simulink model "modules"  (R2017a)
settings: Solver=ode4  StartTime=0.0  StopTime=time_stop  FixedStep=time_step  RelTol=1e-3
values from neighbouring files (symbols this model uses):
  psi = state(3)    [PSVobstacleShip_class.m]    (also in PSVvessel_class.m = obj.eta(3); PsiReferenceModel_class.m = obj.desired_psi_vector; SBMPC_PSVvessel_class.m = obj.eta(3))
undefined symbols (not defined in the file or in its folder): beta, Delta_guidance, Delta_matrix, eta_initial, initial_desired_psi_vector, initial_desired_u_vector, initial_next_waypoint_indexes, initial_obstacle_ship_states, initial_obstacle_ship_states_dot, initial_reference_psi_vector, initial_reference_u_vector, initial_SBMPC_desired_psi_vector, initial_SBMPC_desired_u_vector, initial_SBMPC_next_waypoint_indexes, initial_SBMPC_obstacle_ship_states, initial_SBMPC_obstacle_ship_states_dot, initial_SBMPC_reference_psi_vector, initial_SBMPC_reference_u_vector, initial_SBMPC_x_d_psi_matrix, initial_SBMPC_x_d_u_matrix, initial_state, initial_x_d_psi_matrix, initial_x_d_u_matrix, K_sway, K_yaw, Kp_feedback_linearization, kp_heading, Nmax, nu_initial, num_obs_ship_waypoints, num_prediction_time_steps, number_of_control_behaviors, number_of_obstacle_ships, number_of_SBMPC_obstacle_ships, obs_speed_between_waypoints, obstacle_waypoint_matrix, Omega_matrix, own_ship_reference_psi_init, own_ship_reference_speed, Psi_init, radius_of_acceptance, SBMPC_obs_speed_between_waypoints, SBMPC_obstacle_waypoint_matrix, seconds_between_prediction, state_vector_init, T, T_k_surge, T_k_sway, T_k_yaw, T_s, T_waypoints, time_step, tsamp, U, U_init, V_init, waypoints_obstacle_ships, waypoints_own_ship, Xmax, Ymax
(part 5 of 5)

== matlab function modules/Own-ship/SBMPC /Own-ship trajectory prediction/Own ship trajectory prediction ==
  settings: updateMethod=DISCRETE  sampleTime=time_step
  data: t_0 input; T_s parameter; Kp_feedback_linearization parameter; kp_heading parameter; Xmax parameter; Ymax parameter; Nmax parameter; K_sway parameter; K_yaw parameter; T_k_surge parameter; T_k_sway parameter; T_k_yaw parameter; eta_initial input; nu_initial input; T parameter; Delta_matrix parameter; Omega_matrix parameter; waypoints_matrix input; next_waypoint_index input; own_ship_reference_speed parameter; Delta_guidance parameter; radius_of_acceptance parameter; beta parameter; propulsion_commands parameter; heading_angle_offset_commands parameter; seconds_between_prediction parameter; num_prediction_time_steps parameter; own_ship_x_predicted output size=[num_prediction_time_steps, number_of_control_behaviors]; own_ship_y_predicted output size=[num_prediction_time_steps, number_of_control_behaviors]; own_ship_heading_predicted output size=[num_prediction_time_steps, number_of_control_behaviors]; own_ship_u_predicted output size=[num_prediction_time_steps, number_of_control_behaviors]; own_ship_v_predicted output size=[num_prediction_time_steps, number_of_control_behaviors]; number_of_control_behaviors parameter; own_ship_reference_psi_init parameter
function [own_ship_x_predicted, own_ship_y_predicted, own_ship_heading_predicted, own_ship_u_predicted, own_ship_v_predicted  ]   = ownShipTrajectoryPrediction(t_0, T_s, Kp_feedback_linearization, kp_heading, Xmax, Ymax, Nmax, K_sway, K_yaw, T_k_surge, T_k_sway, T_k_yaw, eta_initial, nu_initial, T, Delta_matrix, Omega_matrix, waypoints_matrix, next_waypoint_index, own_ship_reference_speed, Delta_guidance, radius_of_acceptance, beta, propulsion_commands, heading_angle_offset_commands, seconds_between_prediction, num_prediction_time_steps, number_of_control_behaviors, own_ship_reference_psi_init)  
    %2D zero matrices. One row for each time step in prediction horizon and one column for each control behavior/scenario. 
    own_ship_x_predicted = zeros(num_prediction_time_steps, number_of_control_behaviors);%own_ship_x_predicted_initialization;       
    own_ship_y_predicted = zeros(num_prediction_time_steps, number_of_control_behaviors);%own_ship_y_predicted_initialization;       
    own_ship_heading_predicted = zeros(num_prediction_time_steps, number_of_control_behaviors);%own_ship_heading_predicted_initialization;
    own_ship_u_predicted = zeros(num_prediction_time_steps, number_of_control_behaviors);%own_ship_u_predicted_initialization;
    own_ship_v_predicted = zeros(num_prediction_time_steps, number_of_control_behaviors);%own_ship_v_predicted_initialization;
    
    if (mod(t_0, seconds_between_prediction) == 0)   %only do calculation every "seconds_between_prediction" second.
        psvParameters = coder.load('PSVparameters');
        psvModelParameters = psvParameters.model_config;
        psv_vessel = SBMPC_PSVvessel_class(psvModelParameters, eta_initial, nu_initial, T_s, Kp_feedback_linearization, kp_heading, Xmax, Ymax, Nmax, K_sway, K_yaw, T_k_surge, T_k_sway, T_k_yaw);

        x =  psv_vessel.state(1);
        y =  psv_vessel.state(2);
        vessel_position = [x,y];
        waypointGuidanceObject = SBMPC_waypointGuidance_class(own_ship_reference_psi_init, waypoints_matrix, next_waypoint_index, vessel_position, Delta_guidance, beta, T_s, radius_of_acceptance);              

        scenario_index = 1;  %count for control behaviors
        for Pr = propulsion_commands
            for psi_ca = heading_angle_offset_commands                        
                psv_vessel = psv_vessel.resetPSVState(); %Reset PSV state at start of scenario.
                waypointGuidanceObject = waypointGuidanceObject.resetWaypoints(next_waypoint_index);
                x_d_speed = [nu_initial(1);nu_initial(2);nu_initial(3);0;0;0];
                x_d_heading = [eta_initial(1);eta_initial(2);eta_initial(3);0;0;0;0;0;0];
                for t = 1:num_prediction_time_steps       
                    %Guidance
                    x =  psv_vessel.state(1);
                    y =  psv_vessel.state(2);
                    vessel_position = [x,y];
                    waypointGuidanceObject = waypointGuidanceObject.updateVesselPosition(vessel_position);
                    waypointGuidanceObject = waypointGuidanceObject.updateCurrentWaypoint();                    
                    [waypointGuidanceObject, reference_psi] = waypointGuidanceObject.getReferencePsi();  
                    reference_u = own_ship_reference_speed;

                    %Speed reference model
                    x_d_speed = speedReferenceModel(x_d_speed, reference_u, T_s, Delta_matrix, Omega_matrix);
                    desired_nu = x_d_speed(1:3); 
                    desired_nu(1) = desired_nu(1)*Pr;   %change desired speed in u-direction.
                    
                    x_d_heading = referenceModelPsi(x_d_heading, reference_psi, Omega_matrix, T_s);
                    desired_psi = psi_ca + x_d_heading(3); 
                    

                    [psv_vessel, tau] = psv_vessel.updateStates(desired_psi, desired_nu);       
                    state = psv_vessel.state;                    
                    
                    own_ship_x_predicted(t,scenario_index) = state(1);
                    own_ship_y_predicted(t,scenario_index) = state(2);
                    own_ship_heading_predicted(t,scenario_index) = state(3);
                    own_ship_u_predicted(t,scenario_index) = state(4);
                    own_ship_v_predicted(t,scenario_index) = state(5);
                end %end for
                scenario_index = scenario_index + 1;
            end % end for
        end % end for    
    end %end if    
        
end

== matlab function modules/obstacle ships/Obstacle vessels ==
  data: desired_psi_vector input; desired_u_vector input; obstacle_ships_state_matrix output; X output; Y output; Psi output; U output; V output; R output; Nmax parameter; Ymax parameter; Xmax parameter; kp_heading parameter; Kp_feedback_linearization parameter; initial_obstacle_ship_states parameter; time_step parameter; initial_obstacle_ship_states_dot parameter; number_of_obstacle_ships parameter; K_sway parameter; K_yaw parameter; T_k_yaw parameter; T_k_sway parameter; T_k_surge parameter; state_vector_init parameter; obs_eta output; obs_nu output
function [obstacle_ships_state_matrix, X, Y, Psi, U, V, R, obs_eta, obs_nu] = obstacleVessels(desired_psi_vector, desired_u_vector, Nmax, Ymax, Xmax, kp_heading, Kp_feedback_linearization, initial_obstacle_ship_states, time_step, initial_obstacle_ship_states_dot, number_of_obstacle_ships, K_sway, K_yaw,  T_k_yaw, T_k_sway, T_k_surge, state_vector_init)
    persistent obstacle_ships
    
    if (isempty(obstacle_ships))
        psvParameters = coder.load('PSVparameters');
        psvModelParameters = psvParameters.model_config;
        obstacle_ships = obstacleShips_class(number_of_obstacle_ships, initial_obstacle_ship_states, initial_obstacle_ship_states_dot, desired_psi_vector, desired_u_vector, time_step, psvModelParameters, Kp_feedback_linearization, kp_heading, Xmax, Ymax, Nmax, K_sway, K_yaw, T_k_surge, T_k_sway, T_k_yaw);
    end
    
    
    obstacle_ships = obstacle_ships.updateDesiredSpeedVector(desired_u_vector);
    obstacle_ships = obstacle_ships.updateDesiredPsiVector(desired_psi_vector);    
    obstacle_ships = obstacle_ships.updateObstacleShipsStates();
    
    %each column i in the obstacleShipsStateMatrix is the state [x,y,psi,u,v,r] for obstacle ship number i
    obstacle_ships_state_matrix = obstacle_ships.getObstacleShipsStateMatrix(); 

    
    %column vectors with states. Each element/row r is value for obstacle ship number r
    X = obstacle_ships_state_matrix(1,:);
    Y = obstacle_ships_state_matrix(2,:);
    Psi = obstacle_ships_state_matrix(3,:);
    U = obstacle_ships_state_matrix(4,:);
    V = obstacle_ships_state_matrix(5,:);
    R = obstacle_ships_state_matrix(6,:); 
    obs_eta = [X', Y', Psi'];
    obs_nu  = [U', V', R'];
    
end

== matlab function modules/obstacle ships/find position matrix ==
  data: obstacles_x_position input; position_matrix output; obstacles_y_position input; obstacle_ships_position_matrix_init parameter
function position_matrix = findObstaclePositionMatrix(obstacles_x_position, obstacles_y_position, obstacle_ships_position_matrix_init)
%obstacle positon matrix: %each row r contains x and y position for obstacle ship r

position_matrix = obstacle_ships_position_matrix_init;

position_matrix(:,1) = obstacles_x_position; 
position_matrix(:,2) = obstacles_y_position;
end

== matlab function modules/obstacle ships/guidance /MATLAB Function1 ==
  data: u_vector output; initial_reference_u_vector parameter; next_waypoints_indexes input; obs_speed_between_waypoints parameter; number_of_obstacle_ships parameter
function u_vector = reference_u_vector(initial_reference_u_vector, next_waypoints_indexes, obs_speed_between_waypoints, number_of_obstacle_ships)
    u_vector = initial_reference_u_vector;  %row vector
    for i = 1:number_of_obstacle_ships
        u_vector(i) = obs_speed_between_waypoints(i,next_waypoints_indexes(i)-1);
    end % end for
    
end

== matlab function modules/obstacle ships/guidance /obstacle waypoint guidance ==
  data: obstacle_waypoints input; reference_psi_vector output; state_matrix input; time_step parameter; beta parameter; Delta_guidance parameter; radius_of_acceptance parameter; initial_obstacle_ship_states parameter; number_of_obstacle_ships parameter; initial_reference_psi_vector parameter; initial_next_waypoint_indexes parameter; next_waypoints_indexes output
function [reference_psi_vector, next_waypoints_indexes]  = obstacleWaypointGuidance(obstacle_waypoints, state_matrix, time_step, beta, Delta_guidance, radius_of_acceptance, initial_obstacle_ship_states, number_of_obstacle_ships, initial_reference_psi_vector, initial_next_waypoint_indexes)
    persistent obstaclewaypointGuidanceObject;
    
    if (isempty(obstaclewaypointGuidanceObject))
        obstaclewaypointGuidanceObject = obstacleWaypointGuidance_class(obstacle_waypoints, initial_obstacle_ship_states, Delta_guidance, beta, radius_of_acceptance, time_step, number_of_obstacle_ships, initial_reference_psi_vector, initial_next_waypoint_indexes);
    end
    obstaclewaypointGuidanceObject = obstaclewaypointGuidanceObject.updateObstaclePositions(state_matrix);
    obstaclewaypointGuidanceObject = obstaclewaypointGuidanceObject.updateCurrentWaypoints();
    [obstaclewaypointGuidanceObject, reference_psi_vector] = obstaclewaypointGuidanceObject.getReferencePsiVector();
    next_waypoints_indexes = obstaclewaypointGuidanceObject.getNextWaypointsIndexes();
end

== matlab function modules/obstacle ships/reference model for psi/psi reference model  ==
  data: reference_psi_vector input; desired_psi_vector output; time_step parameter; Delta_matrix parameter; Omega_matrix parameter; initial_reference_psi_vector parameter; number_of_obstacle_ships parameter; initial_desired_psi_vector parameter; initial_x_d_psi_matrix parameter
function desired_psi_vector = obstacleShipsReferenceModelPsi(reference_psi_vector,time_step, Delta_matrix, Omega_matrix, initial_reference_psi_vector,number_of_obstacle_ships,initial_desired_psi_vector, initial_x_d_psi_matrix)

persistent psi_reference_model;

if (isempty(psi_reference_model))
   psi_reference_model = PsiReferenceModel_class(number_of_obstacle_ships, initial_reference_psi_vector, initial_desired_psi_vector, initial_x_d_psi_matrix, Omega_matrix, Delta_matrix, time_step); 
end

psi_reference_model = psi_reference_model.updateReferencePsi(reference_psi_vector);
[psi_reference_model, desired_psi_vector]  = psi_reference_model.updateDesiredPsi();
end

== matlab function modules/obstacle ships/reference model for u/MATLAB Function1 ==
  data: desired_u_vector output; reference_u_vetor input; number_of_obstacle_ships parameter; initial_reference_u_vector parameter; initial_desired_u_vector parameter; initial_x_d_u_matrix parameter; Omega_matrix parameter; Delta_matrix parameter; time_step parameter
function desired_u_vector  = fcn(reference_u_vetor, number_of_obstacle_ships, initial_reference_u_vector, initial_desired_u_vector, initial_x_d_u_matrix, Omega_matrix, Delta_matrix, time_step)
persistent u_reference_model;



if (isempty(u_reference_model))
    u_reference_model = uReferenceModel_class(number_of_obstacle_ships, initial_reference_u_vector, initial_desired_u_vector, initial_x_d_u_matrix, Omega_matrix, Delta_matrix, time_step);
end

u_reference_model = u_reference_model.updateReferenceU(reference_u_vetor);
[u_reference_model, desired_u_vector] = u_reference_model.updateDesiredU();



end

== matlab function modules/SBMPC obstacle ships/SBMPC using intentions /Combine normal obs and own-ship obs ship data  ==
  settings: updateMethod=DISCRETE  sampleTime=time_step
  data: normal_obstacle_ships_x_predicted input size=[number_of_obstacle_ships, num_prediction_time_steps]; obs_x_predicted output size=[1+number_of_obstacle_ships, num_prediction_time_steps]; normal_obstacle_ships_y_predicted input size=[number_of_obstacle_ships, num_prediction_time_steps]; normal_obstacle_ships_Psi input size=[number_of_obstacle_ships, num_prediction_time_steps]; normal_obstacle_ships_U input size=[number_of_obstacle_ships, num_prediction_time_steps]; normal_obsatcle_ships_V input size=[number_of_obstacle_ships, num_prediction_time_steps]; obs_y_predicted output size=[1+number_of_obstacle_ships, num_prediction_time_steps]; obs_psi output size=[1+number_of_obstacle_ships, num_prediction_time_steps]; obs_u output size=[1+number_of_obstacle_ships, num_prediction_time_steps]; obs_v output size=[1+number_of_obstacle_ships, num_prediction_time_steps]; own_ship_obs_x_predicted input size=[num_prediction_time_steps, 1]; own_ship_obs_y_predicted input size=[num_prediction_time_steps, 1]; own_ship_obs_psi input size=[num_prediction_time_steps, 1]; own_ship_obs_u input size=[num_prediction_time_steps, 1]; own_ship_obs_v input size=[num_prediction_time_steps, 1]
function [obs_x_predicted, obs_y_predicted, obs_psi, obs_u, obs_v] = combineNormalAndOwnShipObstacleShipData(normal_obstacle_ships_x_predicted,  normal_obstacle_ships_y_predicted, normal_obstacle_ships_Psi, normal_obstacle_ships_U, normal_obsatcle_ships_V, own_ship_obs_x_predicted, own_ship_obs_y_predicted, own_ship_obs_psi, own_ship_obs_u, own_ship_obs_v)   
   %Data: own ship data as first element , then all normal obstacles data 
   
    obs_x_predicted = [own_ship_obs_x_predicted'; normal_obstacle_ships_x_predicted ];
    obs_y_predicted = [own_ship_obs_y_predicted'; normal_obstacle_ships_y_predicted ];
    
    obs_psi = [own_ship_obs_psi'; normal_obstacle_ships_Psi ]; 
    obs_u   = [own_ship_obs_u';   normal_obstacle_ships_U   ];
    obs_v   = [own_ship_obs_v';   normal_obsatcle_ships_V   ];
   
end

== matlab function modules/Own-ship/SBMPC /Predict obstacle trajectories/Combine normal and SBMPC obstacle ship data  ==
  data: normal_obstacle_ships_x_predicted input size=[num_prediction_time_steps, number_of_obstacle_ships]; obs_x_predicted output size=[num_prediction_time_steps, total_number_of_obstacle_ships]; normal_obstacle_ships_y_predicted input size=[num_prediction_time_steps, number_of_obstacle_ships]; normal_obstacle_ships_Psi input size=[num_prediction_time_steps, number_of_obstacle_ships]; normal_obstacle_ships_U input size=[num_prediction_time_steps, number_of_obstacle_ships]; normal_obsatcle_ships_V input size=[num_prediction_time_steps, number_of_obstacle_ships]; SBMPC_obstacle_ships_X_predicted input size=[number_of_SBMPC_obstacle_ships,num_prediction_time_steps]; SBMPC_obstacle_ships_Y_predicted input size=[number_of_SBMPC_obstacle_ships,num_prediction_time_steps]; SBMPC_obstacle_ships_Psi input size=[number_of_SBMPC_obstacle_ships,num_prediction_time_steps]; SBMPC_obstacle_ships_U input size=[number_of_SBMPC_obstacle_ships,num_prediction_time_steps]; SBMPC_obstacle_ships_V input size=[number_of_SBMPC_obstacle_ships,num_prediction_time_steps]; obs_y_predicted output size=[num_prediction_time_steps, total_number_of_obstacle_ships]; obs_psi output size=[num_prediction_time_steps, total_number_of_obstacle_ships]; obs_u output size=[num_prediction_time_steps, total_number_of_obstacle_ships]; obs_v output size=[num_prediction_time_steps, total_number_of_obstacle_ships]
function [obs_x_predicted, obs_y_predicted, obs_psi, obs_u, obs_v] = combineNormalAndSBMPCObstacleShipData(normal_obstacle_ships_x_predicted,  normal_obstacle_ships_y_predicted, normal_obstacle_ships_Psi, normal_obstacle_ships_U, normal_obsatcle_ships_V,SBMPC_obstacle_ships_X_predicted, SBMPC_obstacle_ships_Y_predicted, SBMPC_obstacle_ships_Psi, SBMPC_obstacle_ships_U, SBMPC_obstacle_ships_V)   
    
    obs_x_predicted = [normal_obstacle_ships_x_predicted, SBMPC_obstacle_ships_X_predicted'];
    obs_y_predicted = [normal_obstacle_ships_y_predicted, SBMPC_obstacle_ships_Y_predicted'];
    
    obs_psi = [normal_obstacle_ships_Psi, SBMPC_obstacle_ships_Psi']; 
    obs_u   = [normal_obstacle_ships_U, SBMPC_obstacle_ships_U'];
    obs_v   = [normal_obsatcle_ships_V, SBMPC_obstacle_ships_V'];
   
end

== matlab function modules/SBMPC obstacle ships/find SBMPC position matrix ==
  data: obstacles_x_position input; position_matrix output; obstacles_y_position input; SBMPC_obstacle_ships_position_matrix_init parameter
function position_matrix = findSBMPCObstaclePositionMatrix(obstacles_x_position, obstacles_y_position, SBMPC_obstacle_ships_position_matrix_init)
%obstacle positon matrix: %each row r contains x and y position for obstacle ship r

position_matrix = SBMPC_obstacle_ships_position_matrix_init;

position_matrix(:,1) = obstacles_x_position; 
position_matrix(:,2) = obstacles_y_position;
end

== matlab function modules/SBMPC obstacle ships/guidance /SBMPC reference u vector ==
  data: u_vector output; initial_SBMPC_reference_u_vector parameter; next_waypoints_indexes input; SBMPC_obs_speed_between_waypoints parameter; number_of_SBMPC_obstacle_ships parameter
function u_vector = reference_u_vector(initial_SBMPC_reference_u_vector, next_waypoints_indexes, SBMPC_obs_speed_between_waypoints, number_of_SBMPC_obstacle_ships)
    u_vector = initial_SBMPC_reference_u_vector;  %row vector
    for i = 1:number_of_SBMPC_obstacle_ships
        u_vector(i) = SBMPC_obs_speed_between_waypoints(i,next_waypoints_indexes(i)-1);
    end % end for
    
end

== matlab function modules/SBMPC obstacle ships/guidance /SBMPC obstacle waypoint guidance ==
  data: SBMPC_obstacle_waypoints input; reference_psi_vector output; state_matrix input; time_step parameter; beta parameter; Delta_guidance parameter; radius_of_acceptance parameter; initial_SBMPC_obstacle_ship_states parameter; number_of_SBMPC_obstacle_ships parameter; initial_SBMPC_reference_psi_vector parameter; initial_SBMPC_next_waypoint_indexes parameter; next_waypoints_indexes output
function [reference_psi_vector, next_waypoints_indexes]  = SBMPCobstacleWaypointGuidance(SBMPC_obstacle_waypoints, state_matrix, time_step, beta, Delta_guidance, radius_of_acceptance, initial_SBMPC_obstacle_ship_states, number_of_SBMPC_obstacle_ships, initial_SBMPC_reference_psi_vector , initial_SBMPC_next_waypoint_indexes)
    persistent obstaclewaypointGuidanceObject;
    
    if (isempty(obstaclewaypointGuidanceObject))
        obstaclewaypointGuidanceObject = obstacleWaypointGuidance_class(SBMPC_obstacle_waypoints, initial_SBMPC_obstacle_ship_states, Delta_guidance, beta, radius_of_acceptance, time_step, number_of_SBMPC_obstacle_ships, initial_SBMPC_reference_psi_vector, initial_SBMPC_next_waypoint_indexes);
    end
    obstaclewaypointGuidanceObject = obstaclewaypointGuidanceObject.updateObstaclePositions(state_matrix);
    obstaclewaypointGuidanceObject = obstaclewaypointGuidanceObject.updateCurrentWaypoints();
    [obstaclewaypointGuidanceObject, reference_psi_vector] = obstaclewaypointGuidanceObject.getReferencePsiVector();
    next_waypoints_indexes = obstaclewaypointGuidanceObject.getNextWaypointsIndexes();
end

== matlab function modules/SBMPC obstacle ships/reference model for psi/SBMPC psi reference model  ==
  data: reference_psi_vector input; desired_psi_vector output; time_step parameter; Delta_matrix parameter; Omega_matrix parameter; initial_SBMPC_reference_psi_vector parameter; number_of_SBMPC_obstacle_ships parameter; initial_SBMPC_desired_psi_vector parameter; initial_SBMPC_x_d_psi_matrix parameter
function desired_psi_vector = SBMPCobstacleShipsReferenceModelPsi(reference_psi_vector,time_step, Delta_matrix, Omega_matrix, initial_SBMPC_reference_psi_vector,number_of_SBMPC_obstacle_ships,initial_SBMPC_desired_psi_vector, initial_SBMPC_x_d_psi_matrix)

persistent psi_reference_model;

if (isempty(psi_reference_model))
   psi_reference_model = PsiReferenceModel_class(number_of_SBMPC_obstacle_ships, initial_SBMPC_reference_psi_vector, initial_SBMPC_desired_psi_vector, initial_SBMPC_x_d_psi_matrix, Omega_matrix, Delta_matrix, time_step); 
end

psi_reference_model = psi_reference_model.updateReferencePsi(reference_psi_vector);
[psi_reference_model, desired_psi_vector]  = psi_reference_model.updateDesiredPsi();


%desired_psi_vector is a row vector

end

== matlab function modules/SBMPC obstacle ships/reference model for u/SBMPC obstacle ships reference model u ==
  data: desired_u_vector output; reference_u_vetor input; number_of_SBMPC_obstacle_ships parameter; initial_SBMPC_reference_u_vector parameter; initial_SBMPC_desired_u_vector parameter; initial_SBMPC_x_d_u_matrix parameter; Omega_matrix parameter; Delta_matrix parameter; time_step parameter
function desired_u_vector  = SBMPCobstacleShipsReferenceModelU(reference_u_vetor, number_of_SBMPC_obstacle_ships, initial_SBMPC_reference_u_vector, initial_SBMPC_desired_u_vector, initial_SBMPC_x_d_u_matrix, Omega_matrix, Delta_matrix, time_step)
persistent u_reference_model;



if (isempty(u_reference_model))
    u_reference_model = uReferenceModel_class(number_of_SBMPC_obstacle_ships, initial_SBMPC_reference_u_vector, initial_SBMPC_desired_u_vector, initial_SBMPC_x_d_u_matrix, Omega_matrix, Delta_matrix, time_step);
end

u_reference_model = u_reference_model.updateReferenceU(reference_u_vetor);
[u_reference_model, desired_u_vector] = u_reference_model.updateDesiredU();

%desired u is a row vector
end

== matlab function modules/SBMPC obstacle ships/SBMPC using intentions /Normal obstacle ships trajectories prediction/Normal obstacle ships trajectories prediction ==
  settings: updateMethod=DISCRETE  sampleTime=time_step
  data: obstacle_ships_psi input; obstacle_ships_u input; obstacle_ships_v input; obstacle_ships_x_predicted output size=[number_of_obstacle_ships, num_prediction_time_steps]; obstacle_ships_y_predicted output size=[number_of_obstacle_ships, num_prediction_time_steps]; obstacle_ships_next_waypoint_index_vector input; obstacle_ships_positions input; T_s parameter; t_0 input; number_of_obstacle_ships parameter; T parameter; seconds_between_prediction parameter; num_prediction_time_steps parameter; num_obs_ship_waypoints parameter; waypoints_obstacle_ships parameter; U parameter; psi parameter; T_waypoints parameter; obstacle_ships_u_predicted output size=[number_of_obstacle_ships, num_prediction_time_steps]; obstacle_ships_v_predicted output size=[number_of_obstacle_ships, num_prediction_time_steps]; obstacle_ships_psi_predicted output size=[number_of_obstacle_ships, num_prediction_time_steps]
function [obstacle_ships_x_predicted,obstacle_ships_y_predicted, obstacle_ships_u_predicted, obstacle_ships_v_predicted, obstacle_ships_psi_predicted] = normalObstacleShipsTrajectoryPrediction(obstacle_ships_psi,obstacle_ships_u, obstacle_ships_v, obstacle_ships_next_waypoint_index_vector, obstacle_ships_positions, T_s, t_0, number_of_obstacle_ships, T, seconds_between_prediction, num_prediction_time_steps, num_obs_ship_waypoints, waypoints_obstacle_ships, U, psi, T_waypoints)
     obstacle_ships_x_predicted   = zeros(number_of_obstacle_ships, num_prediction_time_steps);
     obstacle_ships_y_predicted   = zeros(number_of_obstacle_ships, num_prediction_time_steps);
     obstacle_ships_u_predicted   = zeros(number_of_obstacle_ships, num_prediction_time_steps);
     obstacle_ships_v_predicted   = zeros(number_of_obstacle_ships, num_prediction_time_steps);
     obstacle_ships_psi_predicted = zeros(number_of_obstacle_ships, num_prediction_time_steps);
     if (mod(t_0, seconds_between_prediction) == 0)                 %Only do calculation every "seconds_between_prediction" second.
         for obstacle_ship_index = 1:number_of_obstacle_ships
            obstacle_ships_x_predicted(obstacle_ship_index, 1)   = obstacle_ships_positions(obstacle_ship_index, 1);
            obstacle_ships_y_predicted(obstacle_ship_index, 1)   = obstacle_ships_positions(obstacle_ship_index, 2);
            obstacle_ships_u_predicted(obstacle_ship_index, 1)   = obstacle_ships_u(obstacle_ship_index);
            obstacle_ships_v_predicted(obstacle_ship_index, 1)   = obstacle_ships_v(obstacle_ship_index);
            obstacle_ships_psi_predicted(obstacle_ship_index, 1) = obstacle_ships_psi(obstacle_ship_index);
            for i = 2:num_prediction_time_steps
                obstacle_ship_speed = sqrt((obstacle_ships_u(obstacle_ship_index))^2 + (obstacle_ships_v(obstacle_ship_index))^2);
                obstacle_ships_u_predicted(obstacle_ship_index, i)   = obstacle_ships_u(obstacle_ship_index);
                obstacle_ships_v_predicted(obstacle_ship_index, i)   = obstacle_ships_v(obstacle_ship_index);
                obstacle_ships_psi_predicted(obstacle_ship_index, i) = obstacle_ships_psi(obstacle_ship_index);
                obstacle_ships_x_predicted(obstacle_ship_index, i) =  obstacle_ships_x_predicted(obstacle_ship_index, i-1) + obstacle_ship_speed*cos(obstacle_ships_psi(obstacle_ship_index))*(T_s);
                obstacle_ships_y_predicted(obstacle_ship_index, i) =  obstacle_ships_y_predicted(obstacle_ship_index, i-1) + obstacle_ship_speed*sin(obstacle_ships_psi(obstacle_ship_index))*(T_s);
            end
          
         end % end for
     end % end if

end

== matlab function modules/SBMPC obstacle ships/SBMPC using intentions /SBMPC obstacles: own-ship trajectory prediction/Own ship trajectory prediction ==
  settings: updateMethod=DISCRETE  sampleTime=time_step
  data: t_0 input; T_s parameter; Kp_feedback_linearization parameter; kp_heading parameter; Xmax parameter; Ymax parameter; Nmax parameter; K_sway parameter; K_yaw parameter; T_k_surge parameter; T_k_sway parameter; T_k_yaw parameter; eta_initial input; nu_initial input; T parameter; Delta_matrix parameter; Omega_matrix parameter; waypoints_matrix input; next_waypoint_index input; Delta_guidance parameter; radius_of_acceptance parameter; beta parameter; propulsion_commands parameter; heading_angle_offset_commands parameter; seconds_between_prediction parameter; num_prediction_time_steps parameter; own_ship_x_predicted output size=[number_of_SBMPC_obstacle_ships, num_prediction_time_steps, number_of_control_behaviors]; own_ship_y_predicted output size=[number_of_SBMPC_obstacle_ships, num_prediction_time_steps, number_of_control_behaviors]; own_ship_heading_predicted output size=[number_of_SBMPC_obstacle_ships, num_prediction_time_steps, number_of_control_behaviors]; own_ship_u_predicted output size=[number_of_SBMPC_obstacle_ships, num_prediction_time_steps, number_of_control_behaviors]; own_ship_v_predicted output size=[number_of_SBMPC_obstacle_ships, num_prediction_time_steps, number_of_control_behaviors]; number_of_control_behaviors parameter; SBMPC_obs_speed_between_waypoints parameter; number_of_SBMPC_obstacle_ships parameter; SBMPC_reference_psi_init parameter
function [own_ship_x_predicted, own_ship_y_predicted, own_ship_heading_predicted, own_ship_u_predicted, own_ship_v_predicted  ]   = ownShipTrajectoryPrediction(t_0, T_s, Kp_feedback_linearization, kp_heading, Xmax, Ymax, Nmax, K_sway, K_yaw, T_k_surge, T_k_sway, T_k_yaw, eta_initial, nu_initial, T, Delta_matrix, Omega_matrix, waypoints_matrix, next_waypoint_index, Delta_guidance, radius_of_acceptance, beta, propulsion_commands, heading_angle_offset_commands, seconds_between_prediction, num_prediction_time_steps, number_of_control_behaviors, SBMPC_obs_speed_between_waypoints, number_of_SBMPC_obstacle_ships, SBMPC_reference_psi_init)  
    own_ship_x_predicted       = zeros(number_of_SBMPC_obstacle_ships, num_prediction_time_steps, number_of_control_behaviors); 
    own_ship_y_predicted       = zeros(number_of_SBMPC_obstacle_ships, num_prediction_time_steps, number_of_control_behaviors);   
    own_ship_heading_predicted = zeros(number_of_SBMPC_obstacle_ships, num_prediction_time_steps, number_of_control_behaviors);
    own_ship_u_predicted       = zeros(number_of_SBMPC_obstacle_ships, num_prediction_time_steps, number_of_control_behaviors);
    own_ship_v_predicted       = zeros(number_of_SBMPC_obstacle_ships, num_prediction_time_steps, number_of_control_behaviors);
   
    if (mod(t_0, seconds_between_prediction) == 0)   %only do calculation every "seconds_between_prediction" second.
        for SBMPC_obstacle_ship_index = 1:number_of_SBMPC_obstacle_ships
            psvParameters = coder.load('PSVparameters');
            psvModelParameters = psvParameters.model_config;
            
            SBMPC_obs_eta_initial = eta_initial(SBMPC_obstacle_ship_index,:)';
            SBMPC_obs_nu_initial  = nu_initial(SBMPC_obstacle_ship_index, :)';
            psv_vessel = SBMPC_PSVvessel_class(psvModelParameters, SBMPC_obs_eta_initial, SBMPC_obs_nu_initial, T_s, Kp_feedback_linearization, kp_heading, Xmax, Ymax, Nmax, K_sway, K_yaw, T_k_surge, T_k_sway, T_k_yaw);
            x =  psv_vessel.state(1);
            y =  psv_vessel.state(2);
            vessel_position = [x,y];
            SBMPC_obs_waypoint_matrix = waypoints_matrix(:,:,SBMPC_obstacle_ship_index);
            SBMPC_obs_next_waypoint_index = next_waypoint_index(SBMPC_obstacle_ship_index);            
            
            waypointGuidanceObject = SBMPC_waypointGuidance_class(SBMPC_reference_psi_init(SBMPC_obstacle_ship_index), SBMPC_obs_waypoint_matrix, SBMPC_obs_next_waypoint_index, vessel_position, Delta_guidance, beta, T_s, radius_of_acceptance); 
            
            scenario_index = 1;  %count for control behaviors
            for Pr = propulsion_commands
                for psi_ca = heading_angle_offset_commands 
                    psv_vessel = psv_vessel.resetPSVState(); %Reset PSV state at start of scenario.
                    waypointGuidanceObject = waypointGuidanceObject.resetWaypoints(SBMPC_obs_next_waypoint_index);
                    x_d_speed = [SBMPC_obs_nu_initial(1);SBMPC_obs_nu_initial(2);SBMPC_obs_nu_initial(3);0;0;0];
                    x_d_heading = [SBMPC_obs_eta_initial(1);SBMPC_obs_eta_initial(2);SBMPC_obs_eta_initial(3);0;0;0;0;0;0];
                    for t = 1:num_prediction_time_steps   
                        x =  psv_vessel.state(1);
                        y =  psv_vessel.state(2);
                        vessel_position = [x,y];
                        waypointGuidanceObject = waypointGuidanceObject.updateVesselPosition(vessel_position);
                        waypointGuidanceObject = waypointGuidanceObject.updateCurrentWaypoint();  
                        [waypointGuidanceObject, reference_psi] = waypointGuidanceObject.getReferencePsi();  
                        reference_u   = SBMPC_obs_speed_between_waypoints(SBMPC_obstacle_ship_index, 1);
                        
                        %Speed reference model
                        x_d_speed = speedReferenceModel(x_d_speed, reference_u, T_s, Delta_matrix, Omega_matrix);
                        desired_nu = x_d_speed(1:3); 
                        desired_nu(1) = desired_nu(1)*Pr;   %change desired speed in u-direction.
                        x_d_heading = referenceModelPsi(x_d_heading, reference_psi, Omega_matrix, T_s);
                        desired_psi = psi_ca + x_d_heading(3);
                        
                        [psv_vessel, tau] = psv_vessel.updateStates(desired_psi, desired_nu);  
                        state = psv_vessel.state;                          
                        own_ship_x_predicted(SBMPC_obstacle_ship_index, t, scenario_index) = state(1);
                        own_ship_y_predicted(SBMPC_obstacle_ship_index, t, scenario_index) = state(2);
                        own_ship_heading_predicted(SBMPC_obstacle_ship_index, t, scenario_index) = state(3);
                        own_ship_u_predicted(SBMPC_obstacle_ship_index, t, scenario_index) = state(4);
                        own_ship_v_predicted(SBMPC_obstacle_ship_index, t, scenario_index) = state(5);
                    end % end for
                    scenario_index = scenario_index + 1;
                end % end for
            end % end for  
        end % end for
    end % end if
end

== matlab function modules/SBMPC obstacle ships/Find normal obstacle ships' u, v, psi ==
  data: nu input; normal_obs_U output; eta input; normal_obs_V output; normal_obs_Psi output; number_of_obstacle_ships parameter; U_init parameter; V_init parameter; Psi_init parameter
function [normal_obs_U, normal_obs_V, normal_obs_Psi]  = findNormalObsVariables(nu, eta, number_of_obstacle_ships, U_init, V_init, Psi_init)
    %inpu nu:   contains a  row [u,v,r] for each obstacle
    %input eta: contains a  row [x,y,psi] for each obstacle
    normal_obs_U = U_init;
    normal_obs_V = V_init;
    normal_obs_Psi = Psi_init;
    for i = 1:number_of_obstacle_ships
        normal_obs_U(i) = nu(i, 1);
        normal_obs_V(i) = nu(i, 2);
        normal_obs_Psi(i) = eta(i, 3);
    end

end

== matlab function modules/Own-ship/SBMPC /Find chosen own ship predicted trajectory ==
  data: chosen_scenario_index input; own_ship_x_predicted input size=[num_prediction_time_steps, number_of_control_behaviors]; own_ship_y_predicted input size=[num_prediction_time_steps, number_of_control_behaviors]; chosen_x_predicted output size=[num_prediction_time_steps, 1]; chosen_y_predicted output size=[num_prediction_time_steps, 1]; chosen_psi_predicted output size=[num_prediction_time_steps, 1]; chosen_u_predicted output size=[num_prediction_time_steps, 1]; chosen_v_predicted output size=[num_prediction_time_steps, 1]; own_ship_psi_predicted input size=[num_prediction_time_steps, number_of_control_behaviors]; own_ship_u_predicted input size=[num_prediction_time_steps, number_of_control_behaviors]; own_ship_v_predicted input size=[num_prediction_time_steps, number_of_control_behaviors]
function [chosen_x_predicted, chosen_y_predicted, chosen_psi_predicted, chosen_u_predicted, chosen_v_predicted] = findOwnShipsChosenPredictedTrajectory(chosen_scenario_index, own_ship_x_predicted, own_ship_y_predicted, own_ship_psi_predicted, own_ship_u_predicted, own_ship_v_predicted)


    
    chosen_x_predicted = own_ship_x_predicted(:, chosen_scenario_index);
    chosen_y_predicted = own_ship_y_predicted(:, chosen_scenario_index);
    chosen_psi_predicted = own_ship_psi_predicted(:,chosen_scenario_index);
    chosen_u_predicted = own_ship_u_predicted(:, chosen_scenario_index);
    chosen_v_predicted = own_ship_v_predicted(:, chosen_scenario_index);
end

== matlab function modules/SBMPC obstacle ships/SBMPC using intentions /Find chosen SBMPC obs own ship predicted trajectory ==
  data: chosen_y_predicted output size=[number_of_SBMPC_obstacle_ships,num_prediction_time_steps]; chosen_scenario_index input; own_ship_x_predicted_input input size=[number_of_SBMPC_obstacle_ships, num_prediction_time_steps, number_of_control_behaviors]; own_ship_y_predicted_input input size=[number_of_SBMPC_obstacle_ships, num_prediction_time_steps, number_of_control_behaviors]; own_ship_psi_predicted_input input size=[number_of_SBMPC_obstacle_ships, num_prediction_time_steps, number_of_control_behaviors]; own_ship_u_predicted_input input size=[number_of_SBMPC_obstacle_ships, num_prediction_time_steps, number_of_control_behaviors]; own_ship_v_predicted_input input size=[number_of_SBMPC_obstacle_ships, num_prediction_time_steps, number_of_control_behaviors]; chosen_x_predicted output size=[number_of_SBMPC_obstacle_ships,num_prediction_time_steps]; num_prediction_time_steps parameter; number_of_SBMPC_obstacle_ships parameter; chosen_u_predicted output size=[number_of_SBMPC_obstacle_ships,num_prediction_time_steps]; chosen_v_predicted output size=[number_of_SBMPC_obstacle_ships,num_prediction_time_steps]; chosen_psi_predicted output size=[number_of_SBMPC_obstacle_ships,num_prediction_time_steps]; number_of_control_behaviors parameter
function [chosen_y_predicted, chosen_x_predicted, chosen_u_predicted, chosen_v_predicted, chosen_psi_predicted] = findSBMPCObstacleOwnShipsChosenPredictedTrajectory(chosen_scenario_index, own_ship_x_predicted_input, own_ship_y_predicted_input ,own_ship_psi_predicted_input, own_ship_u_predicted_input, own_ship_v_predicted_input, num_prediction_time_steps, number_of_SBMPC_obstacle_ships, number_of_control_behaviors)
    
    chosen_y_predicted   = zeros(number_of_SBMPC_obstacle_ships, num_prediction_time_steps);
    chosen_x_predicted   = zeros(number_of_SBMPC_obstacle_ships, num_prediction_time_steps);
    chosen_u_predicted   = zeros(number_of_SBMPC_obstacle_ships, num_prediction_time_steps);
    chosen_v_predicted   = zeros(number_of_SBMPC_obstacle_ships, num_prediction_time_steps);
    chosen_psi_predicted = zeros(number_of_SBMPC_obstacle_ships, num_prediction_time_steps);
    
    for SBMPC_obs_index = 1:number_of_SBMPC_obstacle_ships
        chosen_x_predicted(SBMPC_obs_index, :) = own_ship_x_predicted_input(SBMPC_obs_index, :, chosen_scenario_index(SBMPC_obs_index));
        chosen_y_predicted(SBMPC_obs_index, :) = own_ship_y_predicted_input(SBMPC_obs_index, :, chosen_scenario_index(SBMPC_obs_index));
        chosen_u_predicted(SBMPC_obs_index, :) = own_ship_u_predicted_input(SBMPC_obs_index, :, chosen_scenario_index(SBMPC_obs_index));
        chosen_v_predicted(SBMPC_obs_index, :) = own_ship_v_predicted_input(SBMPC_obs_index, :, chosen_scenario_index(SBMPC_obs_index));
        chosen_psi_predicted(SBMPC_obs_index, :) = own_ship_psi_predicted_input(SBMPC_obs_index, :, chosen_scenario_index(SBMPC_obs_index));
    end
end

== matlab function modules/Own-ship/SBMPC /Predict obstacle trajectories/SBMPC obstacle ships trajectories prediction/SBMPC obstacle ships trajectories prediction ==
  settings: updateMethod=DISCRETE  sampleTime=time_step
  data: SBMPC_obstacle_ships_x input; SBMPC_obstacle_ships_x_predicted output size=[number_of_SBMPC_obstacle_ships, num_prediction_time_steps]; SBMPC_obstacle_ships_y_predicted output size=[number_of_SBMPC_obstacle_ships, num_prediction_time_steps]; SBMPC_obstacle_ships_y input; SBMPC_obstacle_ships_psi input; SBMPC_obstacle_ships_u input; SBMPC_obstacle_ships_v input; T_s parameter; t_0 input; number_of_SBMPC_obstacle_ships parameter; seconds_between_prediction parameter; num_prediction_time_steps parameter; SBMPC_obstacle_ships_u_predicted output size=[number_of_SBMPC_obstacle_ships, num_prediction_time_steps]; SBMPC_obstacle_ships_v_predicted output size=[number_of_SBMPC_obstacle_ships, num_prediction_time_steps]; SBMPC_obstacle_ships_psi_predicted output size=[number_of_SBMPC_obstacle_ships, num_prediction_time_steps]
function [SBMPC_obstacle_ships_x_predicted,SBMPC_obstacle_ships_y_predicted, SBMPC_obstacle_ships_u_predicted, SBMPC_obstacle_ships_v_predicted, SBMPC_obstacle_ships_psi_predicted] = normalObstacleShipsTrajectoryPrediction(SBMPC_obstacle_ships_x,SBMPC_obstacle_ships_y, SBMPC_obstacle_ships_psi, SBMPC_obstacle_ships_u, SBMPC_obstacle_ships_v , T_s, t_0, number_of_SBMPC_obstacle_ships, seconds_between_prediction, num_prediction_time_steps)
     SBMPC_obstacle_ships_x_predicted = zeros( number_of_SBMPC_obstacle_ships, num_prediction_time_steps);   
     SBMPC_obstacle_ships_y_predicted = zeros( number_of_SBMPC_obstacle_ships, num_prediction_time_steps);   
     SBMPC_obstacle_ships_u_predicted = zeros( number_of_SBMPC_obstacle_ships, num_prediction_time_steps);
     SBMPC_obstacle_ships_v_predicted = zeros( number_of_SBMPC_obstacle_ships, num_prediction_time_steps);
     SBMPC_obstacle_ships_psi_predicted = zeros( number_of_SBMPC_obstacle_ships, num_prediction_time_steps);
     
     if (mod(t_0, seconds_between_prediction) == 0)                 %Only do calculation every "seconds_between_prediction" second.
         for obstacle_ship_index = 1:number_of_SBMPC_obstacle_ships
             SBMPC_obstacle_ships_x_predicted(obstacle_ship_index, 1)   = SBMPC_obstacle_ships_x(obstacle_ship_index);
             SBMPC_obstacle_ships_y_predicted(obstacle_ship_index, 1)   = SBMPC_obstacle_ships_y(obstacle_ship_index);
             SBMPC_obstacle_ships_u_predicted(obstacle_ship_index, 1)   = SBMPC_obstacle_ships_u(obstacle_ship_index);
             SBMPC_obstacle_ships_v_predicted(obstacle_ship_index, 1)   = SBMPC_obstacle_ships_v(obstacle_ship_index);
             SBMPC_obstacle_ships_psi_predicted(obstacle_ship_index, 1) = SBMPC_obstacle_ships_psi(obstacle_ship_index);
             
             for i = 2:num_prediction_time_steps
                obstacle_ship_speed = sqrt(SBMPC_obstacle_ships_u(obstacle_ship_index)^2 + SBMPC_obstacle_ships_v(obstacle_ship_index)^2);
                SBMPC_obstacle_ships_u_predicted(obstacle_ship_index, i)   = SBMPC_obstacle_ships_u(obstacle_ship_index);
                SBMPC_obstacle_ships_v_predicted(obstacle_ship_index, i)   = SBMPC_obstacle_ships_v(obstacle_ship_index);
                SBMPC_obstacle_ships_psi_predicted(obstacle_ship_index, i) = SBMPC_obstacle_ships_psi(obstacle_ship_index);
                SBMPC_obstacle_ships_x_predicted(obstacle_ship_index, i)   = SBMPC_obstacle_ships_x_predicted(obstacle_ship_index, i-1) + obstacle_ship_speed*cos(SBMPC_obstacle_ships_psi_predicted(obstacle_ship_index, i))*(T_s);
                SBMPC_obstacle_ships_y_predicted(obstacle_ship_index, i)   = SBMPC_obstacle_ships_y_predicted(obstacle_ship_index, i-1) + obstacle_ship_speed*sin(SBMPC_obstacle_ships_psi_predicted(obstacle_ship_index, i))*(T_s);
             end
             
         end % end for
     end % end if

end

== matlab function modules/SBMPC obstacle ships/SBMPC using intentions /own-ship obstacle ships trajectories prediction/Normal obstacle ships trajectories prediction ==
  settings: updateMethod=DISCRETE  sampleTime=time_step
  data: obstacle_ship_psi input; obstacle_ship_u input; obstacle_ship_v input; obstacle_ship_x_predicted output size=[num_prediction_time_steps, 1]; obstacle_ship_y_predicted output size=[num_prediction_time_steps, 1]; obstacle_ship_x input; obstacle_ship_y input; T_s parameter; t_0 input; T parameter; seconds_between_prediction parameter; num_prediction_time_steps parameter; obstacle_ship_u_predicted output size=[num_prediction_time_steps, 1]; obstacle_ship_v_predicted output size=[num_prediction_time_steps, 1]; obstacle_ship_psi_predicted output size=[num_prediction_time_steps, 1]
function [obstacle_ship_x_predicted,obstacle_ship_y_predicted, obstacle_ship_u_predicted, obstacle_ship_v_predicted, obstacle_ship_psi_predicted] = ownShipObstacleShipsTrajectoryPrediction(obstacle_ship_psi,obstacle_ship_u, obstacle_ship_v, obstacle_ship_x,obstacle_ship_y , T_s, t_0,  T, seconds_between_prediction, num_prediction_time_steps)
     obstacle_ship_x_predicted   = zeros(num_prediction_time_steps, 1);
     obstacle_ship_y_predicted   = zeros(num_prediction_time_steps, 1);
     obstacle_ship_u_predicted   = zeros(num_prediction_time_steps, 1);
     obstacle_ship_v_predicted   = zeros(num_prediction_time_steps, 1);
     obstacle_ship_psi_predicted = zeros(num_prediction_time_steps, 1);
     if (mod(t_0, seconds_between_prediction) == 0)                 %Only do calculation every "seconds_between_prediction" second.
        obstacle_ship_x_predicted(1)   = obstacle_ship_x;
        obstacle_ship_y_predicted(1)   = obstacle_ship_y;
        obstacle_ship_u_predicted(1)   = obstacle_ship_u;
        obstacle_ship_v_predicted(1)   = obstacle_ship_v;
        obstacle_ship_psi_predicted(1) = obstacle_ship_psi;
        
        for i=2:num_prediction_time_steps
            obstacle_ship_speed = sqrt(obstacle_ship_u^2 + obstacle_ship_v^2);
            obstacle_ship_x_predicted(i)   = obstacle_ship_x_predicted(i-1) + obstacle_ship_speed*cos(obstacle_ship_psi)*T_s;
            obstacle_ship_y_predicted(i)   = obstacle_ship_y_predicted(i-1) + obstacle_ship_speed*sin(obstacle_ship_psi)*T_s;
            obstacle_ship_u_predicted(i)   = obstacle_ship_u;
            obstacle_ship_v_predicted(i)   = obstacle_ship_v;
            obstacle_ship_psi_predicted(i) = obstacle_ship_psi;
        
        end
          
        
     end % end if

end
